simulink model "Copy_of_jair_architecture"  (R2021a)
settings: Solver=FixedStepAuto  StartTime=0.0  StopTime=Ttotal  FixedStep=Ts  RelTol=1e-3
values from neighbouring files (symbols this model uses):
  drone1_v0 = 20    [main.m]    (also in multi_main.m)
  max_psi = pi/4    (= 0.785398163397)    [main.m]    (also in multi_main.m)
  max_vel = 20    [main.m]    (also in multi_main.m)
  min_psi = -pi/4    (= -0.785398163397)    [main.m]    (also in multi_main.m)
  min_vel = 5    [main.m]    (also in multi_main.m)
  target_psi_dot_amplitude = 0.02    [main.m]    (also in multi_main.m)
  target_psi_dot_frequency = 0.03    [main.m]    (also in multi_main.m)
  target_velocity_amplitude = 0.1    [main.m]    (also in multi_main.m)
  target_velocity_bias = 0    [main.m]    (also in multi_main.m)
  target_velocity_frequency = 0.07    [main.m]    (also in multi_main.m)
  Ts = 1/fs    (= 0.05)    [main.m]    (also in multi_main.m)
  volta = 1    [main.m]    (also in multi_main.m)
settings Model: Creator=migue  LastModifiedBy=migue

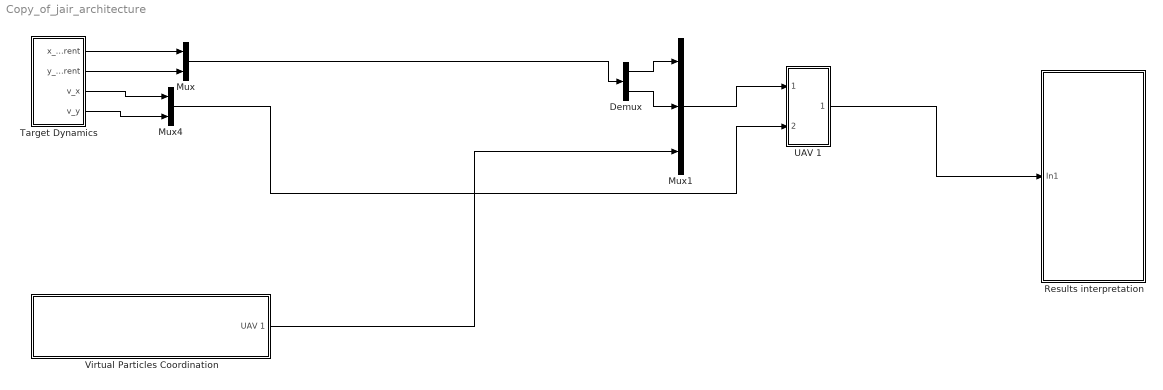
== system Copy_of_jair_architecture ==
  Demux : Demux  Outputs=2
  Mux : Mux  Inputs=2
  Mux1 : Mux  Inputs=3
  Mux4 : Mux  Inputs=2
  Results interpretation : Subsystem
  Target Dynamics : Subsystem
  UAV 1 : Subsystem
  Virtual Particles Coordination : Subsystem
  wires:
  Mux1/1 -> UAV 1/1((x;y))
  UAV 1/1(Out1) -> Results interpretation/1(In1)
  Demux/1 -> Mux1/1
  Demux/2 -> Mux1/2
  Mux/1 -> Demux/1
  Target Dynamics/1(x_current) -> Mux/1
  Target Dynamics/2(y_current) -> Mux/2
  Target Dynamics/3(v_x) -> Mux4/1
  Target Dynamics/4(v_y) -> Mux4/2
  Mux4/1 -> UAV 1/2(Vx e Vy target)
  Virtual Particles Coordination/1(UAV 1) -> Mux1/3

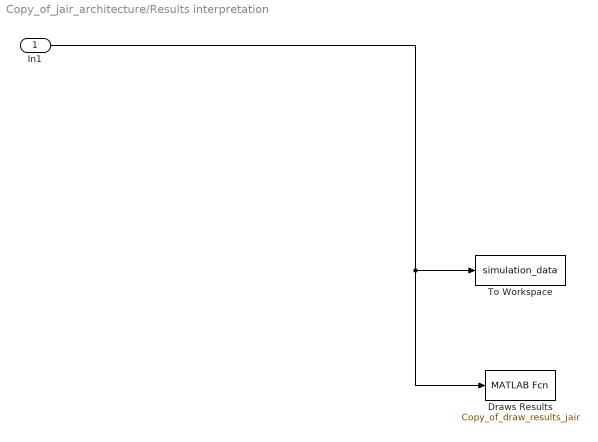
== system Copy_of_jair_architecture/Results interpretation ==
  In1 : Inport
  Draws Results : MATLABFcn  MATLABFcn=Copy_of_draw_results_jair  OutputDimensions=0
  To Workspace : ToWorkspace  VariableName=simulation_data  SampleTime=-1
  wires:
  In1/1 -> Draws Results/1, To Workspace/1

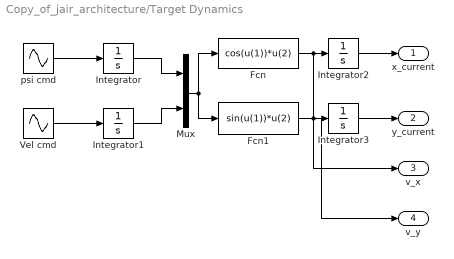
== system Copy_of_jair_architecture/Target Dynamics ==
  Fcn : Fcn  Expr=cos(u(1))*u(2)
  Fcn1 : Fcn  Expr=sin(u(1))*u(2)
  Integrator{,1..3} (4 alike) : Integrator
  Mux : Mux  Inputs=2
  Vel cmd : Sin  Amplitude=target_velocity_amplitude  Bias=target_velocity_bias  Frequency=target_velocity_frequency  SampleTime=Ts
  psi cmd : Sin  Amplitude=target_psi_dot_amplitude  Frequency=target_psi_dot_frequency  Phase=pi/2  SampleTime=Ts
  x_current : Outport  VectorParamsAs1DForOutWhenUnconnected=off
  y_current : Outport  Port=2  VectorParamsAs1DForOutWhenUnconnected=off
  v_x : Outport  Port=3  VectorParamsAs1DForOutWhenUnconnected=off
  v_y : Outport  Port=4  VectorParamsAs1DForOutWhenUnconnected=off
  wires:
  Fcn/1 -> Integrator2/1, v_x/1
  Mux/1 -> Fcn/1, Fcn1/1
  Fcn1/1 -> v_y/1, Integrator3/1
  Integrator3/1 -> y_current/1
  Integrator2/1 -> x_current/1
  psi cmd/1 -> Integrator/1
  Integrator/1 -> Mux/1
  Vel cmd/1 -> Integrator1/1
  Integrator1/1 -> Mux/2

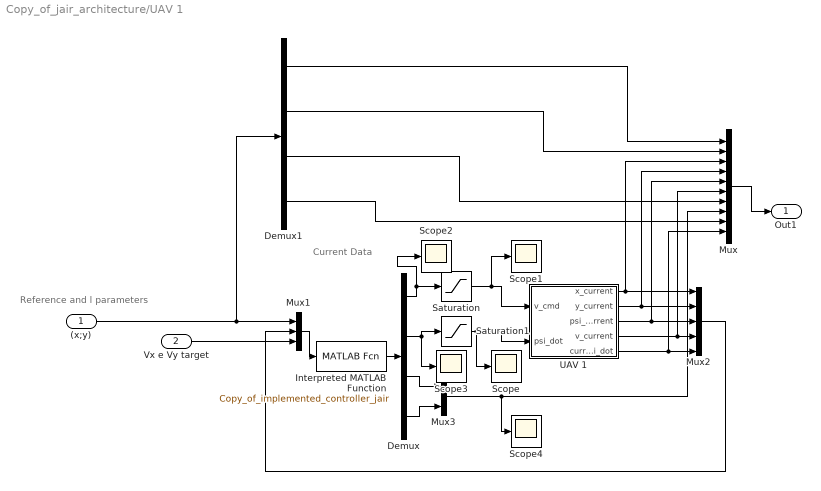
== system Copy_of_jair_architecture/UAV 1 ==
  note: Current Data
  note: Reference and l parameters
  (x;y) : Inport
  Vx e Vy target : Inport  Port=2
  Demux : Demux
  Demux1 : Demux
  Interpreted MATLAB Function : MATLABFcn  MATLABFcn=Copy_of_implemented_controller_jair  OutputDimensions=4
  Mux : Mux  Inputs=10
  Mux1 : Mux  Inputs=3
  Mux2 : Mux  Inputs=5
  Mux3 : Mux  Inputs=2
  Saturation : Saturate  UpperLimit=max_vel  LowerLimit=min_vel
  Saturation1 : Saturate  UpperLimit=max_psi  LowerLimit=min_psi
  Scope{,1..4} (5 alike) : Scope
  UAV 1 : Subsystem
  Out1 : Outport
  wires:
  Mux1/1 -> Interpreted MATLAB Function/1
  Interpreted MATLAB Function/1 -> Demux/1
  Demux/1 -> Scope2/1, Saturation/1
  UAV 1/4(v_current) -> Mux/6, Mux2/4
  Mux2/1 -> Mux1/2
  Demux/2 -> Scope3/1, Saturation1/1
  (x;y)/1 -> Demux1/1, Mux1/1
  Demux1/1 -> Mux/1
  Demux1/2 -> Mux/2
  Mux/1 -> Out1/1
  UAV 1/3(psi_current) -> Mux/5, Mux2/3
  UAV 1/1(x_current) -> Mux/3, Mux2/1
  UAV 1/2(y_current) -> Mux/4, Mux2/2
  UAV 1/5(current_psi_dot) -> Mux/10, Mux2/5
  Saturation/1 -> UAV 1/1(v_cmd), Scope1/1
  Saturation1/1 -> Scope/1, UAV 1/2(psi_dot)
  Mux3/1 -> Scope4/1, Mux/8
  Demux/4 -> Mux3/2
  Demux/3 -> Mux3/1
  Demux1/3 -> Mux/7
  Demux1/4 -> Mux/9
  Vx e Vy target/1 -> Mux1/3

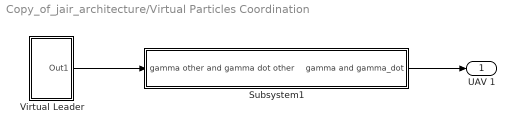
== system Copy_of_jair_architecture/Virtual Particles Coordination ==
  Subsystem1 : Subsystem
  Virtual Leader : Subsystem
  UAV 1 : Outport
  wires:
  Virtual Leader/1(Out1) -> Subsystem1/1(gamma other and gamma dot other)
  Subsystem1/1(gamma and gamma_dot) -> UAV 1/1

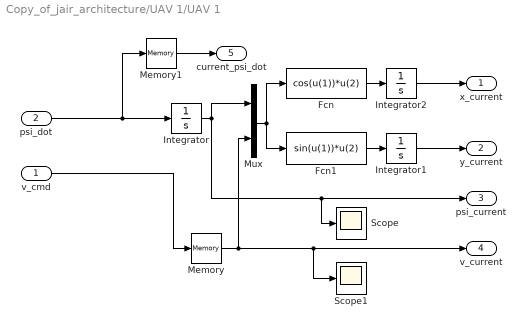
== system Copy_of_jair_architecture/UAV 1/UAV 1 ==
  v_cmd : Inport
  psi_dot : Inport  Port=2
  Fcn : Fcn  Expr=cos(u(1))*u(2)
  Fcn1 : Fcn  Expr=sin(u(1))*u(2)
  Integrator : Integrator
  Integrator1 : Integrator
  Integrator2 : Integrator
  Memory : Memory  InitialCondition=drone1_v0  InheritSampleTime=on
  Memory1 : Memory
  Mux : Mux  Inputs=2
  Scope : Scope
  Scope1 : Scope
  x_current : Outport  VectorParamsAs1DForOutWhenUnconnected=off
  y_current : Outport  Port=2  VectorParamsAs1DForOutWhenUnconnected=off
  psi_current : Outport  Port=3  VectorParamsAs1DForOutWhenUnconnected=off
  v_current : Outport  Port=4  VectorParamsAs1DForOutWhenUnconnected=off
  current_psi_dot : Outport  Port=5
  wires:
  Integrator2/1 -> x_current/1
  Integrator1/1 -> y_current/1
  Fcn/1 -> Integrator2/1
  Fcn1/1 -> Integrator1/1
  Mux/1 -> Fcn/1, Fcn1/1
  v_cmd/1 -> Memory/1
  Integrator/1 -> Mux/1, Scope/1, psi_current/1
  Memory/1 -> Scope1/1, v_current/1, Mux/2
  psi_dot/1 -> Memory1/1, Integrator/1
  Memory1/1 -> current_psi_dot/1

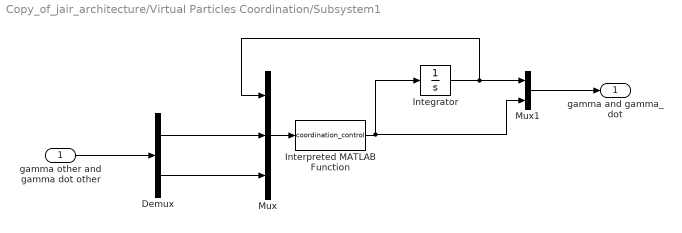
== system Copy_of_jair_architecture/Virtual Particles Coordination/Subsystem1 ==
  gamma other and gamma dot other : Inport
  Demux : Demux  Outputs=2
  Integrator : Integrator
  Interpreted MATLAB Function : MATLABFcn  MATLABFcn=coordination_control  OutputDimensions=1
  Mux : Mux  Inputs=3
  Mux1 : Mux  Inputs=2
  gamma and gamma_dot : Outport
  wires:
  Interpreted MATLAB Function/1 -> Integrator/1, Mux1/2
  Demux/1 -> Mux/2
  Integrator/1 -> Mux1/1, Mux/1
  Mux/1 -> Interpreted MATLAB Function/1
  Mux1/1 -> gamma and gamma_dot/1
  gamma other and gamma dot other/1 -> Demux/1
  Demux/2 -> Mux/3

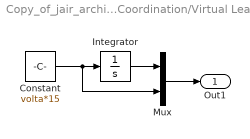
== system Copy_of_jair_architecture/Virtual Particles Coordination/Virtual Leader ==
  Constant : Constant  Value=volta*15
  Integrator : Integrator
  Mux : Mux  Inputs=2
  Out1 : Outport
  wires:
  Mux/1 -> Out1/1
  Integrator/1 -> Mux/1
  Constant/1 -> Integrator/1, Mux/2
